simulink model "open_and_closed_ss_simulink_nl_control101"  (R2025b)
settings: Solver=VariableStepAuto  StartTime=0.0  StopTime=stoptime  RelTol=1e-3
undefined symbols (not defined in the file or in its folder): A, B, C, Ke, Kfbk, x0
settings Model: Creator=Anthony Rossiter  LastModifiedBy=Anthony Rossiter

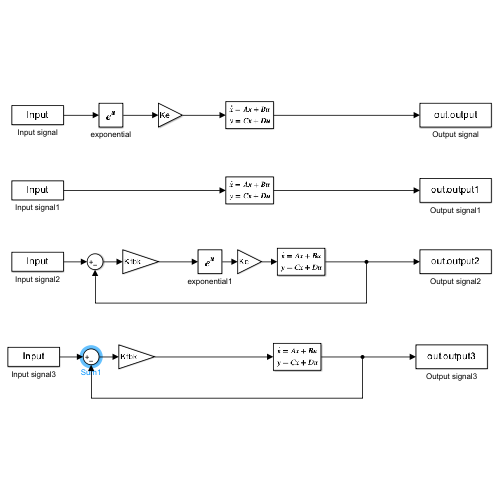
[thumbnail: Simulink's stored preview of the top-level diagram]
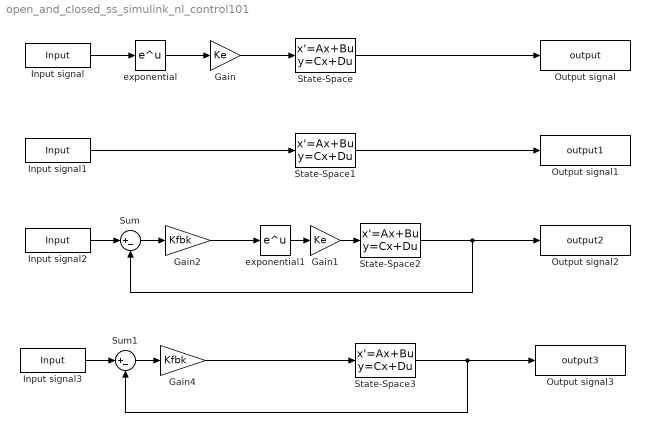
== system open_and_closed_ss_simulink_nl_control101 ==
  Gain : Gain  Gain=Ke
  Gain1 : Gain  Gain=Ke
  Gain2 : Gain  Gain=Kfbk
  Gain4 : Gain  Gain=Kfbk
  Input signal{,1..3} (4 alike) : FromWorkspace  VariableName=Input
  Output signal : ToWorkspace  VariableName=output  SaveFormat=Timeseries  SampleTime=-1
  Output signal1 : ToWorkspace  VariableName=output1  SaveFormat=Timeseries  SampleTime=-1
  Output signal2 : ToWorkspace  VariableName=output2  SaveFormat=Timeseries  SampleTime=-1
  Output signal3 : ToWorkspace  VariableName=output3  SaveFormat=Timeseries  SampleTime=-1
  State-Space{,1..3} (4 alike) : StateSpace  A=A  B=B  C=C  D=0  InitialCondition=x0
  Sum : Sum  Inputs=|+-
  Sum1 : Sum  Inputs=|+-
  exponential : Math
  exponential1 : Math
  wires:
  exponential/1 -> Gain/1
  Input signal/1 -> exponential/1
  State-Space/1 -> Output signal/1
  Gain/1 -> State-Space/1
  State-Space1/1 -> Output signal1/1
  Input signal1/1 -> State-Space1/1
  State-Space2/1 -> Sum/2, Output signal2/1
  exponential1/1 -> Gain1/1
  Gain1/1 -> State-Space2/1
  Input signal2/1 -> Sum/1
  Sum/1 -> Gain2/1
  Gain2/1 -> exponential1/1
  Input signal3/1 -> Sum1/1
  State-Space3/1 -> Sum1/2, Output signal3/1
  Sum1/1 -> Gain4/1
  Gain4/1 -> State-Space3/1
